simulink model "mode_stabilizer_controller"  (R2017a)
settings: Solver=VariableStepAuto  StartTime=0.0  StopTime=inf  RelTol=1e-3
libraries: simulink x1
settings Model: Creator=mini  LastModifiedBy=mini

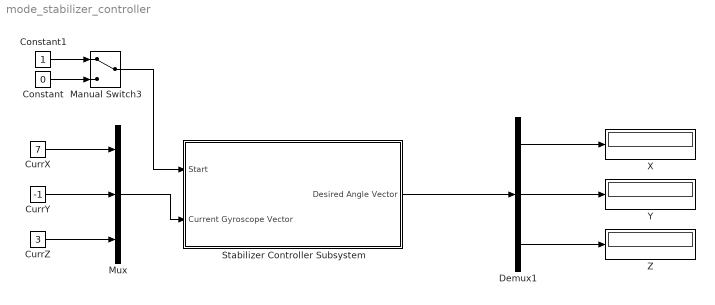
== system mode_stabilizer_controller ==
  Constant : Constant  Value=0
  Constant1 : Constant
  CurrX : Constant  Value=7
  CurrY : Constant  Value=-1
  CurrZ : Constant  Value=3
  Demux1 : Demux  Outputs=3
  Manual Switch3 : ManualSwitch
  Mux : Mux  Inputs=3
  Stabilizer Controller Subsystem : Subsystem
  X : Display
  Y : Display
  Z : Display
  wires:
  Demux1/3 -> Z/1
  Demux1/2 -> Y/1
  Constant/1 -> Manual Switch3/2
  Constant1/1 -> Manual Switch3/1
  Stabilizer Controller Subsystem/1(Desired Angle Vector) -> Demux1/1
  Demux1/1 -> X/1
  Mux/1 -> Stabilizer Controller Subsystem/2(Current Gyroscope Vector)
  CurrX/1 -> Mux/1
  CurrY/1 -> Mux/2
  CurrZ/1 -> Mux/3
  Manual Switch3/1 -> Stabilizer Controller Subsystem/1(Start)

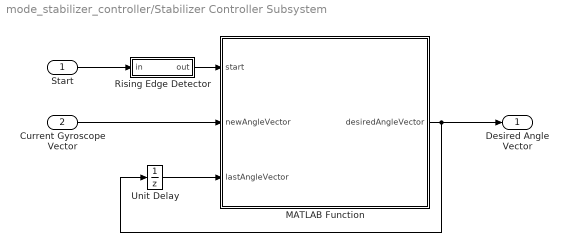
== system mode_stabilizer_controller/Stabilizer Controller Subsystem ==
  Start : Inport
  Current Gyroscope Vector : Inport  Port=2
  MATLAB Function : MATLAB Function  TreatAsAtomicUnit=on
  Rising Edge Detector : Subsystem
  Unit Delay : UnitDelay  SampleTime=-1
  Desired Angle Vector : Outport
  wires:
  Unit Delay/1 -> MATLAB Function/3(lastAngleVector)
  MATLAB Function/1(desiredAngleVector) -> Desired Angle Vector/1, Unit Delay/1
  Current Gyroscope Vector/1 -> MATLAB Function/2(newAngleVector)
  Rising Edge Detector/1(out) -> MATLAB Function/1(start)
  Start/1 -> Rising Edge Detector/1(in)

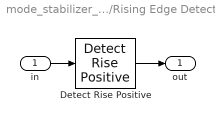
== system mode_stabilizer_controller/Stabilizer Controller Subsystem/Rising Edge Detector ==
  in : Inport  OutDataTypeStr=boolean
  Detect Rise Positive : simulink/Logic and Bit Operations/Detect Rise Positive  vinit=0  OutDataTypeStr=boolean
  out : Outport  OutDataTypeStr=boolean
  wires:
  in/1 -> Detect Rise Positive/1
  Detect Rise Positive/1 -> out/1

== matlab function mode_stabilizer_controller/Stabilizer Controller Subsystem/MATLAB Function ==
  data: start input; newAngleVector input; desiredAngleVector output; lastAngleVector input
function desiredAngleVector = fcn(start, newAngleVector, lastAngleVector)
    % default action on startup 
    if ( start )
        desiredAngleVector = newAngleVector;
    else
        desiredAngleVector = lastAngleVector;
    end
